simulink model "test_SOC_Estim"  (R2021a)
settings: Solver=VariableStepAuto  StartTime=0.0  StopTime=10.0  RelTol=1e-3
settings Model: Creator=miche  LastModifiedBy=miche

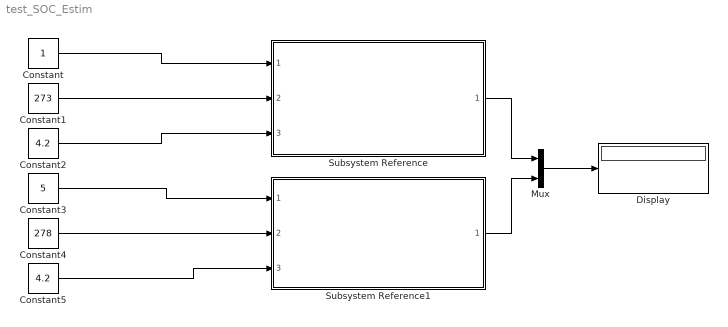
== system test_SOC_Estim ==
  Constant : Constant  OutDataTypeStr=single
  Constant1 : Constant  Value=273  OutDataTypeStr=single
  Constant2 : Constant  Value=4.2  OutDataTypeStr=single
  Constant3 : Constant  Value=5  OutDataTypeStr=single
  Constant4 : Constant  Value=278  OutDataTypeStr=single
  Constant5 : Constant  Value=4.2  OutDataTypeStr=single
  Display : Display
  Mux : Mux  Inputs=2
  Subsystem Reference : Subsystem  ReferencedSubsystem=Single_Cell_SOC_Estimation
  Subsystem Reference1 : Subsystem  ReferencedSubsystem=Single_Cell_SOC_Estimation
  wires:
  Constant/1 -> Subsystem Reference/1
  Constant1/1 -> Subsystem Reference/2
  Constant2/1 -> Subsystem Reference/3
  Subsystem Reference/1 -> Mux/1
  Subsystem Reference1/1 -> Mux/2
  Mux/1 -> Display/1
  Constant3/1 -> Subsystem Reference1/1
  Constant4/1 -> Subsystem Reference1/2
  Constant5/1 -> Subsystem Reference1/3
